simulink model "ControladorContinuo"  (R2020b)
settings: Solver=FixedStepAuto  StartTime=0.0  StopTime=10.0  FixedStep=0.01  RelTol=1e-3
settings Model: Creator=sofia  LastModifiedBy=sofia
settings DataIOCC: SaveOutput=off  SignalLogging=off  DSMLogging=off  SaveTime=off  ReturnWorkspaceOutputs=off

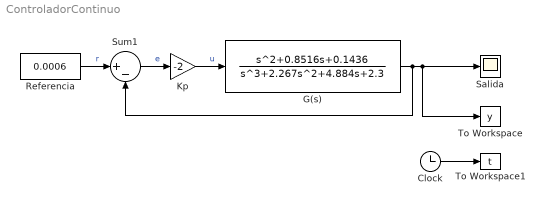
== system ControladorContinuo ==
  Clock : Clock
  G(s) : TransferFcn  Numerator=[1 0.8516 0.1436]  Denominator=[1 2.267 4.884 2.3]
  Kp : Gain  Gain=-2
  Referencia : Constant  Value=0.0006
  Salida : Scope
  Sum1 : Sum  Inputs=|+-
  To Workspace : ToWorkspace  VariableName=y  SampleTime=-1
  To Workspace1 : ToWorkspace  VariableName=t  SampleTime=-1
  wires:
  G(s)/1 -> To Workspace/1, Salida/1, Sum1/2
  Kp/1 -> G(s)/1  "u"
  Sum1/1 -> Kp/1  "e"
  Referencia/1 -> Sum1/1  "r"
  Clock/1 -> To Workspace1/1
